simulink model "model_sim_CHB5_36_new_temp"  (R2020a)
settings: Solver=FixedStepAuto  StartTime=0.0  StopTime=5  RelTol=1e-3
InitFcn:
  | sysinit
values from neighbouring files (symbols this model uses):
  C = 0.03    [sysinit.m]
  C_f = 0.625e-6    (= 6.25e-07)    [sysinit.m]
  f = 50    [sysinit.m]
  f_switch = 500    [sysinit.m]
  L = 0.004    [sysinit.m]
  L_f = 3e-6    (= 3e-06)    [sysinit.m]
  R = 1.2    [sysinit.m]
  R_f = 1.5    [sysinit.m]
  Rth_h = 7.5e-3    (= 0.0075)    [Device_Parameter.m]
  Rth_h_tau = 0.5    [Device_Parameter.m]
  st = 5e-7    (= 5e-07)    [sysinit.m]
  temp_init = 40    [sysinit.m]
  Ts = 1e-6    (= 1e-06)    [sysinit.m]
  Ts2 = 0.5E-3    (= 0.0005)    [sysinit.m]
  Udc = 2500    [sysinit.m]
undefined symbols (not defined in the file or in its folder): DIODE_204520, DIODE_344520, DIODE_D1031SH, DIODE_D1331SH, IGCT_364520_36, IGCT_364521_36, IGCT_654522_6, magnitude, Ts1
libraries: powerlib x278, powerlib_meascontrol x84, simulink x9
(part 1 of 5)
settings Model: SimulationMode=accelerator  Creator=jhchen  LastModifiedBy=Jhchen
settings DataIOCC: ReturnWorkspaceOutputs=off
settings DebuggingCC: UnconnectedInputMsg=none  UnconnectedOutputMsg=none  UnconnectedLineMsg=none
settings ModelReferenceCC: EnableRefExpFcnMdlSchedulingChecks=off
settings RTWCC: Description=Generic Real-Time Target

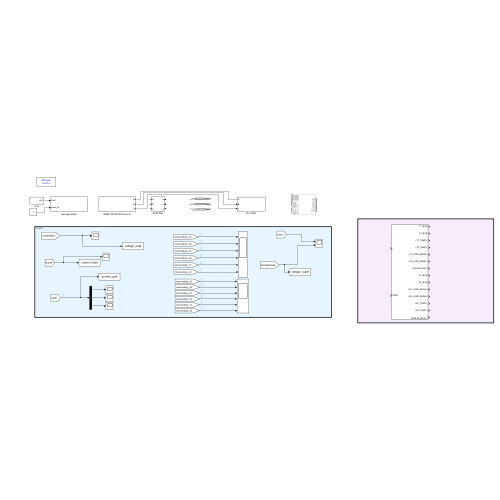
[thumbnail: Simulink's stored preview of the top-level diagram]
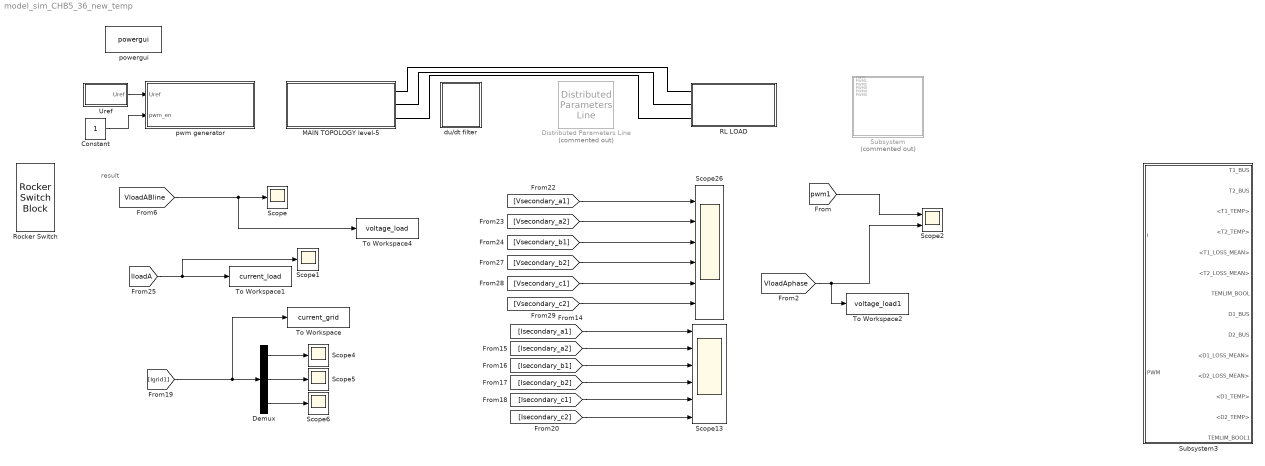
== system model_sim_CHB5_36_new_temp ==
  note: result
  Constant : Constant  OutDataTypeStr=boolean
  Demux : Demux  Outputs=3
  Distributed Parameters Line : powerlib/Elements/Distributed Parameters Line  Commented=on  Phases=3  Length=150e-3  Frequency=60  Resistance=[0.01273 0.3864]  Inductance="[0.9337e-3  4.1264e-3]"  Capacitance=[12.74e-9 7.751e-9]  x1=[0 0 0 0; 0.0001244 0 0 0; 0.0002488 0 0 0; 0.0003733 0 0 0; 0.0004977 0 0 0; 0.0006221 0 0 0]  x2=[0 0 0 0; 0.0001244 0 0 0; 0.0002488 0 0 0; 0.0003733 0 0 0; 0.0004977 0 0 0; 0.0006221 0 0 0]  x3=[0 0 0 0; 0.0001244 0 0 0; 0.0002488 0 0 0; 0.0003733 0 0 0; 0.0004977 0 0 0; 0.0006221 0 0 0]  x4=[0 0 0 0; 0.0001244 0 0 0; 0.0002488 0 0 0; 0.0003733 0 0 0; 0.0004977 0 0 0; 0.0006221 0 0 0]  x5=0  V1=ones(3,3)  V2=ones(3,3)  I1=ones(3,3)  I2=ones(3,3)  nHarmo=1  Measurements=None  Decoupling=off  VsMag0=0  VrMag0=0  VsAngle0=0  VrAngle0=0  IsMag0=0  IrMag0=0  IsAngle0=0  IrAngle0=0
  MAIN TOPOLOGY level-5 : Subsystem
  RL LOAD : Subsystem
  Rocker Switch : RockerSwitchBlock
      settings: Values={{'Off', 'On'}, [0 1]}
  Scope{,1,4..6} (5 alike) : Scope
  Scope13 : Scope  NumInputPorts=6
  Scope2 : Scope  NumInputPorts=2
  Scope26 : Scope  NumInputPorts=6
  Subsystem : Subsystem  Commented=on
  Subsystem3 : Subsystem  mask{IGCTTP=65L4522, DIODE_TP=34L4520}
      mask prompts: IGCTTP "IGCT_DEVICE"; DIODE_TP "DIODE_DEVICE"
      mask TypeOptions IGCTTP: 36L4520 | 36L4521 | 65L4522
      mask TypeOptions DIODE_TP: 20L4520 | 34L4520 | D1031SH | D1331SH
      mask DialogControl ParameterGroupVar Prompt: DEVICE TYPE
  To Workspace : ToWorkspace  VariableName=current_grid  SaveFormat=Structure With Time  SampleTime=-1
  To Workspace1 : ToWorkspace  VariableName=current_load  SaveFormat=Structure With Time  SampleTime=-1
  To Workspace2 : ToWorkspace  VariableName=voltage_load1  SaveFormat=Structure With Time  SampleTime=-1
  To Workspace4 : ToWorkspace  VariableName=voltage_load  SaveFormat=Structure With Time  SampleTime=-1
  Uref : Subsystem  mask{m=1, f=f, nn=0, deg=0}
      mask prompts: m "m_p调制比"; f "f_module输出频率"; nn "电压增加百分量"; deg "电流移相角度"
      mask DialogControl ParameterGroupVar Prompt: 参数
  du/dt filter : Subsystem
  powergui : powerlib/powergui  Priority=1  SimulationMode=Discrete  SampleTime=st  frequency=60  Iterations=50  frequencyindice=50  Pbase=100e6  ErrMax=1e-4  UnitsV=kV  UnitsW=MW  buscounter=0  FunctionMessages=off  echomessages=off  EnableUseOfTLC=off  CurrentSourceSwitches=off  DisableSnubberDevices=off  DisableRonSwitches=off  DisableVfSwitches=off  DisplayEquations=off  AutomaticDiscreteSolvers=off  SolverType=Tustin/Backward Euler (TBE)  Interpol=off  ExternalGateDelay=off  methode=off  Ts=100  x0status=blocks  SPID=on  SwTol=0  HookPort=off  NonlinearTolerance=1e-4  nMaxIteration=100  ContinueOnMaxIteration=off  RestoreLinks=warning  ResistiveCurrentMeasurement=off  Frange=[0:2:500]  Ylog=off  Xlog=on  ShowGrid=off  save=off  variable=ZData  structure=0  ZoomFFT=off  StartTime=0.0  cycles=1  DisplayStyle=1  fundamental=60  FreqAxis=off  MaxFrequency=1000  frequencyindicesteady=1  RmsSteady=1  display=off
  pwm generator : Subsystem  mask{f_car=f_switch, tt=1/4, ttd=0}
      mask prompts: f_car "f_carrier载波频率"; tt "ts载波移相周期"; ttd "td防直通延时"
      mask DialogControl ParameterGroupVar Prompt: 参数
  wires:
  Uref/1(Uref) -> pwm generator/1(Uref)
  [Isecondary_c2] -> Scope13/6
  [Isecondary_b2] -> Scope13/4
  [Isecondary_a2] -> Scope13/2
  Demux/2 -> Scope5/1
  [Vsecondary_b2] -> Scope26/4
  [Vsecondary_b1] -> Scope26/3
  [Isecondary_c1] -> Scope13/5
  [Vsecondary_a1] -> Scope26/1
  Demux/1 -> Scope4/1
  [Isecondary_a1] -> Scope13/1
  Demux/3 -> Scope6/1
  [Vsecondary_c2] -> Scope26/6
  [Igrid1] -> Demux/1, To Workspace/1
  [IloadA] -> Scope1/1, To Workspace1/1
  [Isecondary_b1] -> Scope13/3
  [Vsecondary_c1] -> Scope26/5
  [VloadABline] -> To Workspace4/1, Scope/1
  [Vsecondary_a2] -> Scope26/2
  [pwm1] -> Scope2/1
  [VloadAphase] -> To Workspace2/1, Scope2/2
  Constant/1 -> pwm generator/2(pwm_en)
  connections:
  RL LOAD/LConn1 -- MAIN TOPOLOGY level-5/RConn1
  RL LOAD/LConn2 -- MAIN TOPOLOGY level-5/RConn2
  RL LOAD/LConn3 -- MAIN TOPOLOGY level-5/RConn3

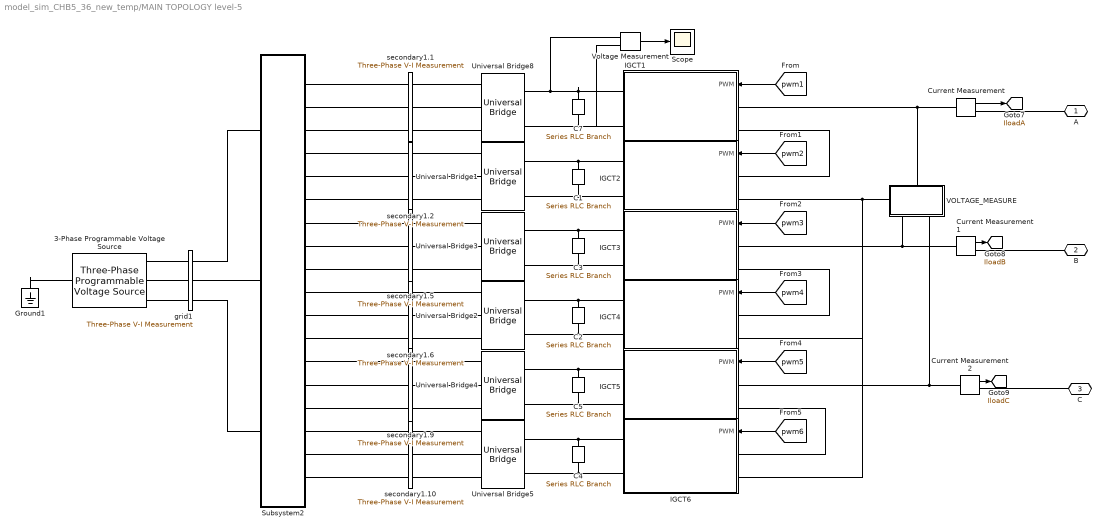
== system model_sim_CHB5_36_new_temp/MAIN TOPOLOGY level-5 ==
  3-Phase Programmable Voltage Source : powerlib/Electrical Sources/Three-Phase Programmable Voltage Source  PositiveSequence=[10000 0 50]  VariationEntity=None  VariationType=Step  VariationTypeAlt=Step  VariationStep=0.5  VariationRate=10  VariationMagnitude=0.3  VariationFrequency=2  VariationTiming=[0.05 1]  VariationPhaseA=off  Amplitudes=[1 0.8 1.2 1.0]  TimeValues=[0 0.1 0.15 0.2]  HarmonicGeneration=off  HarmonicA=[5 0.08 -45 2]  HarmonicB=[2 0 0 2]  Timing="[0.1  1]"  BusType=swing  Pref=0  Qref=0  Qmin=-inf  Qmax=inf
  C{1..5,7} (6 alike) : powerlib/Elements/Series RLC Branch  LConnTagsString=__new0  RConnTagsString=__new0  BranchType=C  Resistance=0.0001  Inductance=1.0  SetiL0=off  InitialCurrent=0  Capacitance=C  Setx0=on  InitialVoltage=2500  Measurements=None
  Current Measurement : powerlib/Measurements/Current Measurement  PhasorSimulation=off  OutputType=Complex  PSBequivalent=0
  Current Measurement1 : powerlib/Measurements/Current Measurement  PhasorSimulation=off  OutputType=Complex  PSBequivalent=0
  Current Measurement2 : powerlib/Measurements/Current Measurement  PhasorSimulation=off  OutputType=Complex  PSBequivalent=0
  Ground1 : powerlib/Elements/Ground  LConnTagsString=a
  IGCT1 : Subsystem
      settings: PortSchema="{\"entries\":[{\"content\":{\"sides\":[{\"content\":{\"connectorIds\":[\"LConn1\",\"LConn2\"]},\"type\":\"ConnectorPlacement.EquallySpacedRectSide\",\"uuid\":\"3b5227fd-32cc-4097-9a6a-2909540651e9\"},{\"content\":{\"connectorIds\":[\"In1\",\"RConn1\",\"RConn2\"],\"side\":\"RIGHT\"},\"type\":\"ConnectorPlacement.EquallySpacedRectSide\",\"uuid\":\"b0068562-9d9a-456b-acd2-db870c5bcace\"},{\"content\":{\"side\":\"TOP\"},\"type\":\"ConnectorPlacement.EquallySpacedRectSide\",\"uuid\":\"bbecbe08-a8e7-4703-9f6f-443f87d924da\"}]},\"type\":\"ConnectorPlacement.EquallySpacedConnector\",\"uuid\":\"6ec83c7b-e3bb-4502-bc8f-4da9ff103a20\"}],\"packageUris\":[\"http://schema.mathworks.com/mf0/Connector/R2020b\"],\"version\":\"1.0\"}"
  IGCT2 : Subsystem
      settings: PortSchema="{\"entries\":[{\"content\":{\"sides\":[{\"content\":{\"connectorIds\":[\"LConn1\",\"LConn2\"]},\"type\":\"ConnectorPlacement.EquallySpacedRectSide\",\"uuid\":\"3b5227fd-32cc-4097-9a6a-2909540651e9\"},{\"content\":{\"connectorIds\":[\"In1\",\"RConn1\",\"RConn2\"],\"side\":\"RIGHT\"},\"type\":\"ConnectorPlacement.EquallySpacedRectSide\",\"uuid\":\"b0068562-9d9a-456b-acd2-db870c5bcace\"},{\"content\":{\"side\":\"TOP\"},\"type\":\"ConnectorPlacement.EquallySpacedRectSide\",\"uuid\":\"bbecbe08-a8e7-4703-9f6f-443f87d924da\"}]},\"type\":\"ConnectorPlacement.EquallySpacedConnector\",\"uuid\":\"6ec83c7b-e3bb-4502-bc8f-4da9ff103a20\"}],\"packageUris\":[\"http://schema.mathworks.com/mf0/Connector/R2020b\"],\"version\":\"1.0\"}"
  IGCT3 : Subsystem
      settings: PortSchema="{\"entries\":[{\"content\":{\"sides\":[{\"content\":{\"connectorIds\":[\"LConn1\",\"LConn2\"]},\"type\":\"ConnectorPlacement.EquallySpacedRectSide\",\"uuid\":\"3b5227fd-32cc-4097-9a6a-2909540651e9\"},{\"content\":{\"connectorIds\":[\"In1\",\"RConn1\",\"RConn2\"],\"side\":\"RIGHT\"},\"type\":\"ConnectorPlacement.EquallySpacedRectSide\",\"uuid\":\"b0068562-9d9a-456b-acd2-db870c5bcace\"},{\"content\":{\"side\":\"TOP\"},\"type\":\"ConnectorPlacement.EquallySpacedRectSide\",\"uuid\":\"bbecbe08-a8e7-4703-9f6f-443f87d924da\"}]},\"type\":\"ConnectorPlacement.EquallySpacedConnector\",\"uuid\":\"6ec83c7b-e3bb-4502-bc8f-4da9ff103a20\"}],\"packageUris\":[\"http://schema.mathworks.com/mf0/Connector/R2020b\"],\"version\":\"1.0\"}"
  IGCT4 : Subsystem
      settings: PortSchema="{\"entries\":[{\"content\":{\"sides\":[{\"content\":{\"connectorIds\":[\"LConn1\",\"LConn2\"]},\"type\":\"ConnectorPlacement.EquallySpacedRectSide\",\"uuid\":\"3b5227fd-32cc-4097-9a6a-2909540651e9\"},{\"content\":{\"connectorIds\":[\"In1\",\"RConn1\",\"RConn2\"],\"side\":\"RIGHT\"},\"type\":\"ConnectorPlacement.EquallySpacedRectSide\",\"uuid\":\"b0068562-9d9a-456b-acd2-db870c5bcace\"},{\"content\":{\"side\":\"TOP\"},\"type\":\"ConnectorPlacement.EquallySpacedRectSide\",\"uuid\":\"bbecbe08-a8e7-4703-9f6f-443f87d924da\"}]},\"type\":\"ConnectorPlacement.EquallySpacedConnector\",\"uuid\":\"6ec83c7b-e3bb-4502-bc8f-4da9ff103a20\"}],\"packageUris\":[\"http://schema.mathworks.com/mf0/Connector/R2020b\"],\"version\":\"1.0\"}"
  IGCT5 : Subsystem
      settings: PortSchema="{\"entries\":[{\"content\":{\"sides\":[{\"content\":{\"connectorIds\":[\"LConn1\",\"LConn2\"]},\"type\":\"ConnectorPlacement.EquallySpacedRectSide\",\"uuid\":\"3b5227fd-32cc-4097-9a6a-2909540651e9\"},{\"content\":{\"connectorIds\":[\"In1\",\"RConn1\",\"RConn2\"],\"side\":\"RIGHT\"},\"type\":\"ConnectorPlacement.EquallySpacedRectSide\",\"uuid\":\"b0068562-9d9a-456b-acd2-db870c5bcace\"},{\"content\":{\"side\":\"TOP\"},\"type\":\"ConnectorPlacement.EquallySpacedRectSide\",\"uuid\":\"bbecbe08-a8e7-4703-9f6f-443f87d924da\"}]},\"type\":\"ConnectorPlacement.EquallySpacedConnector\",\"uuid\":\"6ec83c7b-e3bb-4502-bc8f-4da9ff103a20\"}],\"packageUris\":[\"http://schema.mathworks.com/mf0/Connector/R2020b\"],\"version\":\"1.0\"}"
  IGCT6 : Subsystem
      settings: PortSchema="{\"entries\":[{\"content\":{\"sides\":[{\"content\":{\"connectorIds\":[\"LConn1\",\"LConn2\"]},\"type\":\"ConnectorPlacement.EquallySpacedRectSide\",\"uuid\":\"3b5227fd-32cc-4097-9a6a-2909540651e9\"},{\"content\":{\"connectorIds\":[\"In1\",\"RConn1\",\"RConn2\"],\"side\":\"RIGHT\"},\"type\":\"ConnectorPlacement.EquallySpacedRectSide\",\"uuid\":\"b0068562-9d9a-456b-acd2-db870c5bcace\"},{\"content\":{\"side\":\"TOP\"},\"type\":\"ConnectorPlacement.EquallySpacedRectSide\",\"uuid\":\"bbecbe08-a8e7-4703-9f6f-443f87d924da\"}]},\"type\":\"ConnectorPlacement.EquallySpacedConnector\",\"uuid\":\"6ec83c7b-e3bb-4502-bc8f-4da9ff103a20\"}],\"packageUris\":[\"http://schema.mathworks.com/mf0/Connector/R2020b\"],\"version\":\"1.0\"}"
  Scope : Scope
  Subsystem2 : Subsystem  mask{p=4e6, vp=10000/6, vs=1900, windingpri=[0.0125 0.01], windingsec=[0.0125  0.08], mag=[500  500]}
      mask prompts: p "Nominal power"; vp "Primary nominal voltage Vp (VrmsPh-Ph)"; vs "Scecondary nominal voltage"; windingpri "Winding primary [R L]"; windingsec "Winding secondary [R L]"; mag "Magnetizing branch [Rm Lm]"
      mask DialogControl ParameterGroupVar Prompt: 参数
  Universal Bridge{1..5,8} (6 alike) : powerlib/Power Electronics/Universal Bridge  Arms=3  SnubberResistance=1e5  SnubberCapacitance=inf  Device=Diodes  Ron=1e-3  Lon=0  ForwardVoltages="[  0  0  ]"  ForwardVoltage=0  GTOparameters=[ 10e-6 , 20e-6 ]  IGBTparameters=[ 1e-6 , 2e-6 ]  Measurements=All voltages and currents  Measurements_2=None  converterType=Rectifier
  VOLTAGE_MEASURE : Subsystem
      settings: PortSchema="{\"entries\":[{\"content\":{\"sides\":[{\"content\":{\"connectorIds\":[\"LConn1\"]},\"type\":\"ConnectorPlacement.EquallySpacedRectSide\",\"uuid\":\"e0cdf748-1c1e-4377-bca6-4a33d23f4a26\"},{\"content\":{\"side\":\"RIGHT\"},\"type\":\"ConnectorPlacement.EquallySpacedRectSide\",\"uuid\":\"7345d1e9-e146-4d05-bc9d-06c5f4bfd43e\"},{\"content\":{\"connectorIds\":[\"LConn2\"],\"side\":\"TOP\"},\"type\":\"ConnectorPlacement.EquallySpacedRectSide\",\"uuid\":\"2ef5394b-e3d5-43ec-bd76-ec9d8d58d678\"},{\"content\":{\"connectorIds\":[\"RConn1\",\"RConn2\"],\"side\":\"BOTTOM\"},\"type\":\"ConnectorPlacement.EquallySpacedRectSide\",\"uuid\":\"2dd50293-b78e-4e40-a029-347d4d381fe9\"}]},\"type\":\"ConnectorPlacement.EquallySpacedConnector\",\"uuid\":\"a79e479b-e54c-4d34-8e2f-a0f7c0fb898b\"}],\"packageUris\":[\"http://schema.mathworks.com/mf0/Connector/R2020b\"],\"version\":\"1.0\"}"
  Voltage Measurement : powerlib/Measurements/Voltage Measurement  PhasorSimulation=off  OutputType=Complex  PSBequivalent=0
  grid1 : powerlib/Measurements/Three-Phase V-I Measurement  VoltageMeasurement=phase-to-ground  SetLabelV=on  LabelV=Vgrid1  Vpu=off  VpuLL=off  CurrentMeasurement=yes  SetLabelI=on  LabelI=Igrid1  Ipu=off  Pbase=1e3  Vbase=380  OutputType=Magnitude  PhasorSimulation=off  PSBequivalent=0
  secondary1.1 : powerlib/Measurements/Three-Phase V-I Measurement  VoltageMeasurement=phase-to-phase  SetLabelV=on  LabelV=Vsecondary_a1  Vpu=off  VpuLL=off  CurrentMeasurement=yes  SetLabelI=on  LabelI=Isecondary_a1  Ipu=off  Pbase=1e3  Vbase=380  OutputType=Magnitude  PhasorSimulation=off  PSBequivalent=0
  secondary1.10 : powerlib/Measurements/Three-Phase V-I Measurement  VoltageMeasurement=phase-to-phase  SetLabelV=on  LabelV=Vsecondary_c2  Vpu=off  VpuLL=off  CurrentMeasurement=yes  SetLabelI=on  LabelI=Isecondary_c2  Ipu=off  Pbase=1e3  Vbase=380  OutputType=Magnitude  PhasorSimulation=off  PSBequivalent=0
  secondary1.2 : powerlib/Measurements/Three-Phase V-I Measurement  VoltageMeasurement=phase-to-phase  SetLabelV=on  LabelV=Vsecondary_a2  Vpu=off  VpuLL=off  CurrentMeasurement=yes  SetLabelI=on  LabelI=Isecondary_a2  Ipu=off  Pbase=1e3  Vbase=380  OutputType=Magnitude  PhasorSimulation=off  PSBequivalent=0
  secondary1.5 : powerlib/Measurements/Three-Phase V-I Measurement  VoltageMeasurement=phase-to-phase  SetLabelV=on  LabelV=Vsecondary_b1  Vpu=off  VpuLL=off  CurrentMeasurement=yes  SetLabelI=on  LabelI=Isecondary_b1  Ipu=off  Pbase=1e3  Vbase=380  OutputType=Magnitude  PhasorSimulation=off  PSBequivalent=0
  secondary1.6 : powerlib/Measurements/Three-Phase V-I Measurement  VoltageMeasurement=phase-to-phase  SetLabelV=on  LabelV=Vsecondary_b2  Vpu=off  VpuLL=off  CurrentMeasurement=yes  SetLabelI=on  LabelI=Isecondary_b2  Ipu=off  Pbase=1e3  Vbase=380  OutputType=Magnitude  PhasorSimulation=off  PSBequivalent=0
  secondary1.9 : powerlib/Measurements/Three-Phase V-I Measurement  VoltageMeasurement=phase-to-phase  SetLabelV=on  LabelV=Vsecondary_c1  Vpu=off  VpuLL=off  CurrentMeasurement=yes  SetLabelI=on  LabelI=Isecondary_c1  Ipu=off  Pbase=1e3  Vbase=380  OutputType=Magnitude  PhasorSimulation=off  PSBequivalent=0
  A : PMIOPort  Side=Right
  B : PMIOPort  Port=2  Side=Right
  C : PMIOPort  Port=3  Side=Right
  tag scope: IloadA=global, IloadB=global, IloadC=global
  wires:
  [pwm1] -> IGCT1/1(PWM)
  Current Measurement2/1 -> [IloadC]
  [pwm2] -> IGCT2/1(PWM)
  [pwm5] -> IGCT5/1(PWM)
  [pwm6] -> IGCT6/1(PWM)
  [pwm4] -> IGCT4/1(PWM)
  [pwm3] -> IGCT3/1(PWM)
  Current Measurement1/1 -> [IloadB]
  Current Measurement/1 -> [IloadA]
  Voltage Measurement/1 -> Scope/1
  connections:
  Subsystem2/RConn7 -- secondary1.5/LConn1
  Universal Bridge5/RConn1 -- IGCT6/LConn1 -- C4/LConn1
  Universal Bridge4/LConn2 -- secondary1.9/RConn2
  Current Measurement2/LConn1 -- IGCT5/RConn1 -- VOLTAGE_MEASURE/RConn2
  secondary1.2/RConn1 -- Universal Bridge1/LConn1
  Universal Bridge5/LConn2 -- secondary1.10/RConn2
  Universal Bridge3/RConn1 -- IGCT3/LConn1 -- C3/LConn1
  Subsystem2/RConn5 -- secondary1.2/LConn2
  Ground1/LConn1 -- 3-Phase Programmable Voltage Source/LConn1
  Subsystem2/RConn16 -- secondary1.10/LConn1
  Subsystem2/RConn14 -- secondary1.9/LConn2
  Subsystem2/RConn3 -- secondary1.1/LConn3
  Subsystem2/RConn6 -- secondary1.2/LConn3
  Universal Bridge4/RConn2 -- IGCT5/LConn2 -- C5/RConn1
  Universal Bridge1/RConn1 -- C1/LConn1 -- IGCT2/LConn1
  Current Measurement/LConn1 -- IGCT1/RConn1 -- VOLTAGE_MEASURE/LConn2
  Universal Bridge3/RConn2 -- IGCT3/LConn2 -- C3/RConn1
  Universal Bridge2/RConn1 -- IGCT4/LConn1 -- C2/LConn1
  C7/LConn1 -- IGCT1/LConn1 -- Voltage Measurement/LConn1 -- Universal Bridge8/RConn1
  Universal Bridge1/RConn2 -- IGCT2/LConn2 -- C1/RConn1
  Subsystem2/RConn12 -- secondary1.6/LConn3
  Subsystem2/LConn2 -- grid1/RConn2
  Subsystem2/LConn3 -- grid1/RConn3
  Current Measurement1/LConn1 -- IGCT3/RConn1 -- VOLTAGE_MEASURE/RConn1
  IGCT4/RConn1 -- IGCT3/RConn2
  Subsystem2/RConn15 -- secondary1.9/LConn3
  Universal Bridge5/RConn2 -- IGCT6/LConn2 -- C4/RConn1
  secondary1.2/RConn2 -- Universal Bridge1/LConn2
  C7/RConn1 -- Voltage Measurement/LConn2 -- IGCT1/LConn2 -- Universal Bridge8/RConn2
  secondary1.6/RConn2 -- Universal Bridge2/LConn2
  Universal Bridge4/LConn3 -- secondary1.9/RConn3
  Subsystem2/RConn1 -- secondary1.1/LConn1
  secondary1.1/RConn2 -- Universal Bridge8/LConn2
  grid1/LConn1 -- 3-Phase Programmable Voltage Source/RConn1
  Subsystem2/RConn10 -- secondary1.6/LConn1
  secondary1.1/RConn3 -- Universal Bridge8/LConn3
  grid1/LConn2 -- 3-Phase Programmable Voltage Source/RConn2
  Universal Bridge5/LConn3 -- secondary1.10/RConn3
  Universal Bridge4/LConn1 -- secondary1.9/RConn1
  Universal Bridge5/LConn1 -- secondary1.10/RConn1
  grid1/LConn3 -- 3-Phase Programmable Voltage Source/RConn3
  secondary1.1/RConn1 -- Universal Bridge8/LConn1
  Subsystem2/RConn2 -- secondary1.1/LConn2
  Subsystem2/RConn4 -- secondary1.2/LConn1
  Subsystem2/LConn1 -- grid1/RConn1
  secondary1.6/RConn1 -- Universal Bridge2/LConn1
  secondary1.6/RConn3 -- Universal Bridge2/LConn3
  Universal Bridge2/RConn2 -- IGCT4/LConn2 -- C2/RConn1
  Subsystem2/RConn18 -- secondary1.10/LConn3
  Subsystem2/RConn13 -- secondary1.9/LConn1
  Subsystem2/RConn9 -- secondary1.5/LConn3
  Subsystem2/RConn11 -- secondary1.6/LConn2
  Subsystem2/RConn8 -- secondary1.5/LConn2
  Subsystem2/RConn17 -- secondary1.10/LConn2
  Universal Bridge4/RConn1 -- IGCT5/LConn1 -- C5/LConn1
  IGCT6/RConn1 -- IGCT5/RConn2
  IGCT2/RConn1 -- IGCT1/RConn2
  secondary1.5/RConn2 -- Universal Bridge3/LConn2
  secondary1.5/RConn3 -- Universal Bridge3/LConn3
  secondary1.5/RConn1 -- Universal Bridge3/LConn1
  secondary1.2/RConn3 -- Universal Bridge1/LConn3
  Current Measurement2/RConn1 -- C/RConn1
  Current Measurement/RConn1 -- A/RConn1
  B/RConn1 -- Current Measurement1/RConn1
  IGCT6/RConn2 -- IGCT4/RConn2 -- IGCT2/RConn2 -- VOLTAGE_MEASURE/LConn1

== system model_sim_CHB5_36_new_temp/RL LOAD ==
  Scope : Scope  NumInputPorts=2
  Series RLC Branch1 : powerlib/Elements/Series RLC Branch  LConnTagsString=__new0  RConnTagsString=__new0  BranchType=RL  Resistance=R  Inductance=L  SetiL0=off  InitialCurrent=0  Capacitance=1e-6  Setx0=off  InitialVoltage=0  Measurements=None
  Series RLC Branch2 : powerlib/Elements/Series RLC Branch  LConnTagsString=__new0  RConnTagsString=__new0  BranchType=RL  Resistance=R  Inductance=L  SetiL0=off  InitialCurrent=0  Capacitance=1e-6  Setx0=off  InitialVoltage=0  Measurements=None
  Series RLC Branch7 : powerlib/Elements/Series RLC Branch  LConnTagsString=__new0  RConnTagsString=__new0  BranchType=RL  Resistance=R  Inductance=L  SetiL0=off  InitialCurrent=0  Capacitance=1e-6  Setx0=off  InitialVoltage=0  Measurements=None
  Voltage Measurement : powerlib/Measurements/Voltage Measurement  PhasorSimulation=off  OutputType=Complex  PSBequivalent=0
  A : PMIOPort  Side=Left
  B : PMIOPort  Port=2  Side=Left
  C : PMIOPort  Port=3  Side=Left
  wires:
  Voltage Measurement/1 -> Scope/2
  [VloadAphase] -> Scope/1
  connections:
  Series RLC Branch7/RConn1 -- Series RLC Branch2/RConn1 -- Series RLC Branch1/RConn1 -- Voltage Measurement/LConn2
  Series RLC Branch2/LConn1 -- C/RConn1
  Series RLC Branch7/LConn1 -- Voltage Measurement/LConn1 -- A/RConn1
  Series RLC Branch1/LConn1 -- B/RConn1

== system model_sim_CHB5_36_new_temp/Subsystem ==
  PWM : Inport
  PWM1 : Inport  Port=2
  PWM2 : Inport  Port=3
  PWM3 : Inport  Port=4
  PWM4 : Inport  Port=5
  PWM5 : Inport  Port=6
  IGCT1 : Subsystem
      settings: PortSchema="{\"entries\":[{\"content\":{\"sides\":[{\"content\":{\"connectorIds\":[\"LConn1\",\"LConn2\"]},\"type\":\"ConnectorPlacement.EquallySpacedRectSide\",\"uuid\":\"3b5227fd-32cc-4097-9a6a-2909540651e9\"},{\"content\":{\"connectorIds\":[\"In1\",\"RConn1\",\"RConn2\"],\"side\":\"RIGHT\"},\"type\":\"ConnectorPlacement.EquallySpacedRectSide\",\"uuid\":\"b0068562-9d9a-456b-acd2-db870c5bcace\"},{\"content\":{\"side\":\"TOP\"},\"type\":\"ConnectorPlacement.EquallySpacedRectSide\",\"uuid\":\"bbecbe08-a8e7-4703-9f6f-443f87d924da\"},{\"content\":{\"side\":\"BOTTOM\"},\"type\":\"ConnectorPlacement.EquallySpacedRectSide\",\"uuid\":\"38988ce8-647b-48d0-a974-68b7c64b6edd\"}]},\"type\":\"ConnectorPlacement.EquallySpacedConnector\",\"uuid\":\"6ec83c7b-e3bb-4502-bc8f-4da9ff103a20\"}],\"packageUris\":[\"http://schema.mathworks.com/mf0/Connector/R2020b\"],\"version\":\"1.0\"}"
  IGCT2 : Subsystem
      settings: PortSchema="{\"entries\":[{\"content\":{\"sides\":[{\"content\":{\"connectorIds\":[\"LConn1\",\"LConn2\"]},\"type\":\"ConnectorPlacement.EquallySpacedRectSide\",\"uuid\":\"3b5227fd-32cc-4097-9a6a-2909540651e9\"},{\"content\":{\"connectorIds\":[\"In1\",\"RConn1\",\"RConn2\"],\"side\":\"RIGHT\"},\"type\":\"ConnectorPlacement.EquallySpacedRectSide\",\"uuid\":\"b0068562-9d9a-456b-acd2-db870c5bcace\"},{\"content\":{\"side\":\"TOP\"},\"type\":\"ConnectorPlacement.EquallySpacedRectSide\",\"uuid\":\"bbecbe08-a8e7-4703-9f6f-443f87d924da\"},{\"content\":{\"side\":\"BOTTOM\"},\"type\":\"ConnectorPlacement.EquallySpacedRectSide\",\"uuid\":\"38988ce8-647b-48d0-a974-68b7c64b6edd\"}]},\"type\":\"ConnectorPlacement.EquallySpacedConnector\",\"uuid\":\"6ec83c7b-e3bb-4502-bc8f-4da9ff103a20\"}],\"packageUris\":[\"http://schema.mathworks.com/mf0/Connector/R2020b\"],\"version\":\"1.0\"}"
  IGCT3 : Subsystem
      settings: PortSchema="{\"entries\":[{\"content\":{\"sides\":[{\"content\":{\"connectorIds\":[\"LConn1\",\"LConn2\"]},\"type\":\"ConnectorPlacement.EquallySpacedRectSide\",\"uuid\":\"3b5227fd-32cc-4097-9a6a-2909540651e9\"},{\"content\":{\"connectorIds\":[\"In1\",\"RConn1\",\"RConn2\"],\"side\":\"RIGHT\"},\"type\":\"ConnectorPlacement.EquallySpacedRectSide\",\"uuid\":\"b0068562-9d9a-456b-acd2-db870c5bcace\"},{\"content\":{\"side\":\"TOP\"},\"type\":\"ConnectorPlacement.EquallySpacedRectSide\",\"uuid\":\"bbecbe08-a8e7-4703-9f6f-443f87d924da\"},{\"content\":{\"side\":\"BOTTOM\"},\"type\":\"ConnectorPlacement.EquallySpacedRectSide\",\"uuid\":\"38988ce8-647b-48d0-a974-68b7c64b6edd\"}]},\"type\":\"ConnectorPlacement.EquallySpacedConnector\",\"uuid\":\"6ec83c7b-e3bb-4502-bc8f-4da9ff103a20\"}],\"packageUris\":[\"http://schema.mathworks.com/mf0/Connector/R2020b\"],\"version\":\"1.0\"}"
  IGCT4 : Subsystem
      settings: PortSchema="{\"entries\":[{\"content\":{\"sides\":[{\"content\":{\"connectorIds\":[\"LConn1\",\"LConn2\"]},\"type\":\"ConnectorPlacement.EquallySpacedRectSide\",\"uuid\":\"3b5227fd-32cc-4097-9a6a-2909540651e9\"},{\"content\":{\"connectorIds\":[\"In1\",\"RConn1\",\"RConn2\"],\"side\":\"RIGHT\"},\"type\":\"ConnectorPlacement.EquallySpacedRectSide\",\"uuid\":\"b0068562-9d9a-456b-acd2-db870c5bcace\"},{\"content\":{\"side\":\"TOP\"},\"type\":\"ConnectorPlacement.EquallySpacedRectSide\",\"uuid\":\"bbecbe08-a8e7-4703-9f6f-443f87d924da\"},{\"content\":{\"side\":\"BOTTOM\"},\"type\":\"ConnectorPlacement.EquallySpacedRectSide\",\"uuid\":\"38988ce8-647b-48d0-a974-68b7c64b6edd\"}]},\"type\":\"ConnectorPlacement.EquallySpacedConnector\",\"uuid\":\"6ec83c7b-e3bb-4502-bc8f-4da9ff103a20\"}],\"packageUris\":[\"http://schema.mathworks.com/mf0/Connector/R2020b\"],\"version\":\"1.0\"}"
  IGCT5 : Subsystem
      settings: PortSchema="{\"entries\":[{\"content\":{\"sides\":[{\"content\":{\"connectorIds\":[\"LConn1\",\"LConn2\"]},\"type\":\"ConnectorPlacement.EquallySpacedRectSide\",\"uuid\":\"3b5227fd-32cc-4097-9a6a-2909540651e9\"},{\"content\":{\"connectorIds\":[\"In1\",\"RConn1\",\"RConn2\"],\"side\":\"RIGHT\"},\"type\":\"ConnectorPlacement.EquallySpacedRectSide\",\"uuid\":\"b0068562-9d9a-456b-acd2-db870c5bcace\"},{\"content\":{\"side\":\"TOP\"},\"type\":\"ConnectorPlacement.EquallySpacedRectSide\",\"uuid\":\"bbecbe08-a8e7-4703-9f6f-443f87d924da\"},{\"content\":{\"side\":\"BOTTOM\"},\"type\":\"ConnectorPlacement.EquallySpacedRectSide\",\"uuid\":\"38988ce8-647b-48d0-a974-68b7c64b6edd\"}]},\"type\":\"ConnectorPlacement.EquallySpacedConnector\",\"uuid\":\"6ec83c7b-e3bb-4502-bc8f-4da9ff103a20\"}],\"packageUris\":[\"http://schema.mathworks.com/mf0/Connector/R2020b\"],\"version\":\"1.0\"}"
  IGCT6 : Subsystem
      settings: PortSchema="{\"entries\":[{\"content\":{\"sides\":[{\"content\":{\"connectorIds\":[\"LConn1\",\"LConn2\"]},\"type\":\"ConnectorPlacement.EquallySpacedRectSide\",\"uuid\":\"3b5227fd-32cc-4097-9a6a-2909540651e9\"},{\"content\":{\"connectorIds\":[\"In1\",\"RConn1\",\"RConn2\"],\"side\":\"RIGHT\"},\"type\":\"ConnectorPlacement.EquallySpacedRectSide\",\"uuid\":\"b0068562-9d9a-456b-acd2-db870c5bcace\"},{\"content\":{\"side\":\"TOP\"},\"type\":\"ConnectorPlacement.EquallySpacedRectSide\",\"uuid\":\"bbecbe08-a8e7-4703-9f6f-443f87d924da\"},{\"content\":{\"side\":\"BOTTOM\"},\"type\":\"ConnectorPlacement.EquallySpacedRectSide\",\"uuid\":\"38988ce8-647b-48d0-a974-68b7c64b6edd\"}]},\"type\":\"ConnectorPlacement.EquallySpacedConnector\",\"uuid\":\"6ec83c7b-e3bb-4502-bc8f-4da9ff103a20\"}],\"packageUris\":[\"http://schema.mathworks.com/mf0/Connector/R2020b\"],\"version\":\"1.0\"}"
  Udc+ : PMIOPort  Side=Left
  p1 : PMIOPort  Port=2  Side=Right
  udc- : PMIOPort  Port=3  Side=Left
  p2 : PMIOPort  Port=4  Side=Right
  Udc+1 : PMIOPort  Port=5  Side=Left
  p3 : PMIOPort  Port=6  Side=Right
  udc-1 : PMIOPort  Port=7  Side=Left
  p4 : PMIOPort  Port=8  Side=Right
  Udc+2 : PMIOPort  Port=9  Side=Left
  p5 : PMIOPort  Port=10  Side=Right
  udc-2 : PMIOPort  Port=11  Side=Left
  p6 : PMIOPort  Port=12  Side=Right
  Udc+3 : PMIOPort  Port=13  Side=Left
  p7 : PMIOPort  Port=14  Side=Right
  udc-3 : PMIOPort  Port=15  Side=Left
  p8 : PMIOPort  Port=16  Side=Right
  Udc+4 : PMIOPort  Port=17  Side=Left
  p9 : PMIOPort  Port=18  Side=Right
  udc-4 : PMIOPort  Port=19  Side=Left
  p10 : PMIOPort  Port=20  Side=Right
  Udc+5 : PMIOPort  Port=21  Side=Left
  p11 : PMIOPort  Port=22  Side=Right
  udc-5 : PMIOPort  Port=23  Side=Left
  p12 : PMIOPort  Port=24  Side=Right
  wires:
  PWM/1 -> IGCT1/1(PWM)
  PWM4/1 -> IGCT5/1(PWM)
  PWM3/1 -> IGCT4/1(PWM)
  PWM5/1 -> IGCT6/1(PWM)
  PWM1/1 -> IGCT2/1(PWM)
  PWM2/1 -> IGCT3/1(PWM)
  connections:
  IGCT5/LConn2 -- udc-4/RConn1
  IGCT6/LConn2 -- udc-5/RConn1
  IGCT6/RConn2 -- p12/RConn1
  IGCT6/RConn1 -- p11/RConn1
  IGCT1/LConn1 -- Udc+/RConn1
  IGCT1/LConn2 -- udc-/RConn1
  IGCT6/LConn1 -- Udc+5/RConn1
  IGCT1/RConn1 -- p1/RConn1
  IGCT5/RConn1 -- p9/RConn1
  IGCT2/LConn2 -- udc-1/RConn1
  IGCT3/RConn1 -- p5/RConn1
  IGCT3/RConn2 -- p6/RConn1
  IGCT3/LConn1 -- Udc+2/RConn1
  IGCT2/RConn1 -- p3/RConn1
  IGCT3/LConn2 -- udc-2/RConn1
  IGCT2/RConn2 -- p4/RConn1
  IGCT4/LConn1 -- Udc+3/RConn1
  IGCT4/LConn2 -- udc-3/RConn1
  IGCT5/RConn2 -- p10/RConn1
  IGCT5/LConn1 -- Udc+4/RConn1
  IGCT4/RConn1 -- p7/RConn1
  IGCT4/RConn2 -- p8/RConn1
  IGCT1/RConn2 -- p2/RConn1
  IGCT2/LConn1 -- Udc+1/RConn1

== system model_sim_CHB5_36_new_temp/Subsystem3 ==
  i : Inport
  PWM : Inport  Port=2
  DIODE : Subsystem  Variant=on
  Demux : Demux
  IGCT : Subsystem  Variant=on  VariantControl=Variant Subsystem
  T1_BUS : Outport
  T2_BUS : Outport  Port=2
  <T1_TEMP> : Outport  Port=3
  <T2_TEMP> : Outport  Port=4
  <T1_LOSS_MEAN> : Outport  Port=5
  <T2_LOSS_MEAN> : Outport  Port=6
  TEMLIM_BOOL : Outport  Port=7
  D1_BUS : Outport  Port=8
  D2_BUS : Outport  Port=9
  <D1_LOSS_MEAN> : Outport  Port=10
  <D2_LOSS_MEAN> : Outport  Port=11
  <D1_TEMP> : Outport  Port=12
  <D2_TEMP> : Outport  Port=13
  TEMLIM_BOOL1 : Outport  Port=14
  wires:
  IGCT/2(T2_BUS) -> T2_BUS/1
  DIODE/7(TEMLIM_BOOL) -> TEMLIM_BOOL1/1
  Demux/1 -> DIODE/2(PWM1), IGCT/2(PWM1)
  DIODE/2(D2_BUS) -> D2_BUS/1
  DIODE/3(D1_LOSS_MEAN) -> <D1_LOSS_MEAN>/1
  Demux/2 -> DIODE/3(PWM2), IGCT/3(PWM2)
  Demux/4 -> DIODE/5(PWM4)
  Demux/3 -> DIODE/4(PWM3)
  IGCT/3(<T1_TEMP>) -> <T1_TEMP>/1
  DIODE/6(D2_TEMP) -> <D2_TEMP>/1
  IGCT/1(T1_BUS) -> T1_BUS/1
  IGCT/4(<T2_TEMP>) -> <T2_TEMP>/1
  IGCT/5(<T1_LOSS_MEAN>) -> <T1_LOSS_MEAN>/1
  i/1 -> DIODE/1(I), IGCT/1(I)
  IGCT/6(<T2_LOSS_MEAN>) -> <T2_LOSS_MEAN>/1
  IGCT/7(TEMLIM_BOOL) -> TEMLIM_BOOL/1
  DIODE/5(D1_TEMP) -> <D1_TEMP>/1
  DIODE/4(D2_LOSS_MEAN) -> <D2_LOSS_MEAN>/1
  DIODE/1(D1_BUS) -> D1_BUS/1
  PWM/1 -> Demux/1

== system model_sim_CHB5_36_new_temp/Uref ==
  Mux : Mux  Inputs=3
  Saddle_Wave : Subsystem
  Sine Wave -2/3pi rad : Sin  Amplitude=m*1000*(1+nn)  Frequency=f*2*pi  Phase=-2/3*pi+deg*pi  SampleTime=0
  Sine Wave 0 rad : Sin  Amplitude=m*1000*(1+nn)  Frequency=f*2*pi  Phase=deg*pi  SampleTime=0
  Sine Wave 2/3pi rad : Sin  Amplitude=m*1000*(1+nn)  Frequency=f*2*pi  Phase=2/3*pi+deg*pi  SampleTime=0
  Uref : Outport
  wires:
  Sine Wave 2/3pi rad/1 -> Saddle_Wave/3(C)
  Saddle_Wave/2(b) -> Mux/2
  Saddle_Wave/1(a) -> Mux/1
  Sine Wave 0 rad/1 -> Saddle_Wave/1(A)
  Saddle_Wave/3(c) -> Mux/3
  Sine Wave -2/3pi rad/1 -> Saddle_Wave/2(B)
  Mux/1 -> Uref/1

== system model_sim_CHB5_36_new_temp/du//dt filter ==
  Series RLC Branch1 : powerlib/Elements/Series RLC Branch  LConnTagsString=__new0  RConnTagsString=__new0  BranchType=RC  Resistance=R_f  Inductance=L  SetiL0=off  InitialCurrent=0  Capacitance=C_f  Setx0=off  InitialVoltage=0  Measurements=None
  Series RLC Branch2 : powerlib/Elements/Series RLC Branch  LConnTagsString=__new0  RConnTagsString=__new0  BranchType=RC  Resistance=R_f  Inductance=L  SetiL0=off  InitialCurrent=0  Capacitance=C_f  Setx0=off  InitialVoltage=0  Measurements=None
  Series RLC Branch3 : powerlib/Elements/Series RLC Branch  LConnTagsString=__new0  RConnTagsString=__new0  BranchType=L  Resistance=R  Inductance=L_f  SetiL0=off  InitialCurrent=0  Capacitance=1e-6  Setx0=off  InitialVoltage=0  Measurements=None
  Series RLC Branch4 : powerlib/Elements/Series RLC Branch  LConnTagsString=__new0  RConnTagsString=__new0  BranchType=L  Resistance=R  Inductance=L_f  SetiL0=off  InitialCurrent=0  Capacitance=1e-6  Setx0=off  InitialVoltage=0  Measurements=None
  Series RLC Branch5 : powerlib/Elements/Series RLC Branch  LConnTagsString=__new0  RConnTagsString=__new0  BranchType=L  Resistance=R  Inductance=L_f  SetiL0=off  InitialCurrent=0  Capacitance=1e-6  Setx0=off  InitialVoltage=0  Measurements=None
  Series RLC Branch6 : powerlib/Elements/Series RLC Branch  LConnTagsString=__new0  RConnTagsString=__new0  BranchType=RC  Resistance=R_f  Inductance=L  SetiL0=off  InitialCurrent=0  Capacitance=C_f  Setx0=off  InitialVoltage=0  Measurements=None
  A : PMIOPort  Side=Left
  B : PMIOPort  Port=2  Side=Left
  C : PMIOPort  Port=3  Side=Left
  a : PMIOPort  Port=4  Side=Right
  b : PMIOPort  Port=5  Side=Right
  c : PMIOPort  Port=6  Side=Right
  connections:
  Series RLC Branch5/RConn1 -- C/RConn1
  Series RLC Branch6/LConn1 -- a/RConn1 -- Series RLC Branch3/LConn1
  Series RLC Branch5/LConn1 -- Series RLC Branch2/LConn1 -- c/RConn1
  Series RLC Branch2/RConn1 -- Series RLC Branch6/RConn1 -- Series RLC Branch1/RConn1
  Series RLC Branch1/LConn1 -- b/RConn1 -- Series RLC Branch4/LConn1
  Series RLC Branch4/RConn1 -- B/RConn1
  Series RLC Branch3/RConn1 -- A/RConn1

== system model_sim_CHB5_36_new_temp/pwm generator ==
  Uref : Inport
  pwm_en : Inport  Port=2
  Demux : Demux  Outputs=3
  NOT{1..6} (6 alike) : Logic  AllPortsSameDT=off  OutDataTypeStr=boolean
  Scope1 : Scope  NumInputPorts=4
  carrier : Subsystem
  pwm generator : Subsystem
  pwm generator1 : Subsystem
  pwm generator2 : Subsystem
  tag scope: pwm1=global, pwm2=global, pwm3=global, pwm4=global, pwm5=global, pwm6=global
  wires:
  pwm generator2/1(pwm_up) -> NOT2/1
  pwm generator2/2(pwm_down) -> NOT1/1
  pwm generator1/1(pwm_up) -> NOT4/1
  pwm generator1/2(pwm_down) -> NOT3/1
  pwm generator/1(pwm_up) -> NOT6/1
  pwm generator/2(pwm_down) -> NOT5/1
  Demux/1 -> Scope1/2, pwm generator/1(modulate_wave)
  Demux/2 -> pwm generator1/1(modulate_wave), Scope1/3
  Demux/3 -> Scope1/4, pwm generator2/1(modulate_wave)
  carrier/1(CARRIER_4*1) -> pwm generator2/2(Carrier_wave), pwm generator1/2(Carrier_wave), pwm generator/2(Carrier_wave), Scope1/1
  Uref/1 -> Demux/1
  NOT6/1 -> [pwm1]
  NOT5/1 -> [pwm2]
  NOT4/1 -> [pwm3]
  NOT3/1 -> [pwm4]
  NOT2/1 -> [pwm5]
  NOT1/1 -> [pwm6]
  pwm_en/1 -> NOT1/2, NOT2/2, NOT3/2, NOT4/2, NOT5/2, NOT6/2

== system model_sim_CHB5_36_new_temp/MAIN TOPOLOGY level-5/IGCT1 ==
  PWM : Inport
  Current Measurement1 : powerlib/Measurements/Current Measurement  PhasorSimulation=off  OutputType=Complex  PSBequivalent=0
  Demux : Demux
  Diode{1..3,6,8} (5 alike) : powerlib/Power Electronics/Diode  Ron=rto  Lon=0  Vf=vto  IC=0  UseSnubber=off  Rs=500  Cs=250e-9  Measurements=on
  IGBT{,1..3} (4 alike) : powerlib/Power Electronics/IGBT  Ron=rt  Lon=0  Vf=vt  Tf=1e-6  Tt=2e-6  IC=0  Rs=1e5  Cs=inf  Measurements=on
  Series RLC Branch1 : powerlib/Elements/Series RLC Branch  LConnTagsString=__new0  RConnTagsString=__new0  BranchType=RL  Resistance=1e-5  Inductance=3.0E-6  SetiL0=off  InitialCurrent=0  Capacitance=1e-6  Setx0=off  InitialVoltage=0  Measurements=None
  Series RLC Branch10 : powerlib/Elements/Series RLC Branch  LConnTagsString=__new0  RConnTagsString=__new0  BranchType=L  Resistance=1  Inductance=0.4e-6  SetiL0=off  InitialCurrent=0  Capacitance=1e-6  Setx0=off  InitialVoltage=0  Measurements=None
  Series RLC Branch12 : powerlib/Elements/Series RLC Branch  LConnTagsString=__new0  RConnTagsString=__new0  BranchType=RL  Resistance=1e-5  Inductance=1E-9  SetiL0=off  InitialCurrent=0  Capacitance=1e-6  Setx0=off  InitialVoltage=0  Measurements=None
  Series RLC Branch14 : powerlib/Elements/Series RLC Branch  LConnTagsString=__new0  RConnTagsString=__new0  BranchType=L  Resistance=1  Inductance=1E-7  SetiL0=off  InitialCurrent=0  Capacitance=1e-6  Setx0=off  InitialVoltage=0  Measurements=None
  Series RLC Branch2 : powerlib/Elements/Series RLC Branch  LConnTagsString=__new0  RConnTagsString=__new0  BranchType=RC  Resistance=1e-5  Inductance=20e-6  SetiL0=off  InitialCurrent=0  Capacitance=17e-6  Setx0=off  InitialVoltage=0  Measurements=None
  Series RLC Branch3 : powerlib/Elements/Series RLC Branch  LConnTagsString=__new0  RConnTagsString=__new0  BranchType=RL  Resistance=1e-5  Inductance=1E-9  SetiL0=off  InitialCurrent=0  Capacitance=1e-6  Setx0=off  InitialVoltage=0  Measurements=None
  Series RLC Branch5 : powerlib/Elements/Series RLC Branch  LConnTagsString=__new0  RConnTagsString=__new0  BranchType=L  Resistance=1  Inductance=1E-7  SetiL0=off  InitialCurrent=0  Capacitance=1e-6  Setx0=off  InitialVoltage=0  Measurements=None
  Series RLC Branch7 : powerlib/Elements/Series RLC Branch  LConnTagsString=__new0  RConnTagsString=__new0  BranchType=RL  Resistance=0.6  Inductance=1e-6  SetiL0=off  InitialCurrent=0  Capacitance=1e-6  Setx0=off  InitialVoltage=0  Measurements=None
  Series RLC Branch9 : powerlib/Elements/Series RLC Branch  LConnTagsString=__new0  RConnTagsString=__new0  BranchType=L  Resistance=1  Inductance=0.4e-6  SetiL0=off  InitialCurrent=0  Capacitance=1e-6  Setx0=off  InitialVoltage=0  Measurements=None
  Terminator{,1..9} (10 alike) : Terminator
  Udc+ : PMIOPort  Side=Left
  udc- : PMIOPort  Port=2  Side=Left
  p1 : PMIOPort  Port=3  Side=Right
  p2 : PMIOPort  Port=4  Side=Right
  wires:
  Diode3/1 -> Terminator9/1
  IGBT3/1 -> Terminator5/1
  [n1] -> IGBT3/1
  IGBT1/1 -> Terminator4/1
  IGBT2/1 -> Terminator3/1
  IGBT/1 -> Terminator2/1
  [n2] -> IGBT1/1
  [p1] -> IGBT2/1
  Current Measurement1/1 -> Terminator/1
  Diode2/1 -> Terminator8/1
  [p2] -> IGBT/1
  Diode8/1 -> Terminator7/1
  Diode1/1 -> Terminator6/1
  Diode6/1 -> Terminator1/1
  Demux/3 -> [n2]
  PWM/1 -> Demux/1
  Demux/1 -> [p2]
  Demux/2 -> [p1]
  Demux/4 -> [n1]
  connections:
  Series RLC Branch10/LConn1 -- udc-/RConn1
  Series RLC Branch9/LConn1 -- Udc+/RConn1
  Diode6/RConn1 -- Series RLC Branch7/RConn1 -- Series RLC Branch2/LConn1
  Current Measurement1/LConn1 -- Series RLC Branch1/RConn1 -- Series RLC Branch3/LConn1 -- Series RLC Branch12/LConn1
  Diode3/LConn1 -- IGBT3/RConn1 -- Series RLC Branch14/RConn1
  Series RLC Branch3/RConn1 -- IGBT/LConn1 -- Diode8/RConn1
  Diode1/LConn1 -- Series RLC Branch5/RConn1 -- IGBT1/RConn1
  Current Measurement1/RConn1 -- Diode6/LConn1
  Diode2/RConn1 -- Series RLC Branch12/RConn1 -- IGBT2/LConn1
  p1/RConn1 -- Diode2/LConn1 -- Diode3/RConn1 -- IGBT3/LConn1 -- IGBT2/RConn1
  Series RLC Branch5/LConn1 -- Series RLC Branch14/LConn1 -- Series RLC Branch10/RConn1 -- Series RLC Branch2/RConn1
  Series RLC Branch1/LConn1 -- Series RLC Branch7/LConn1 -- Series RLC Branch9/RConn1
  p2/RConn1 -- IGBT1/LConn1 -- Diode1/RConn1 -- Diode8/LConn1 -- IGBT/RConn1

== system model_sim_CHB5_36_new_temp/MAIN TOPOLOGY level-5/IGCT2 ==
  PWM : Inport
  Current Measurement1 : powerlib/Measurements/Current Measurement  PhasorSimulation=off  OutputType=Complex  PSBequivalent=0
  Demux : Demux
  Diode{1..3,6,8} (5 alike) : powerlib/Power Electronics/Diode  Ron=rto  Lon=0  Vf=vto  IC=0  UseSnubber=off  Rs=500  Cs=250e-9  Measurements=on
  IGBT{,1..3} (4 alike) : powerlib/Power Electronics/IGBT  Ron=rt  Lon=0  Vf=vt  Tf=1e-6  Tt=2e-6  IC=0  Rs=1e5  Cs=inf  Measurements=on
  Series RLC Branch1 : powerlib/Elements/Series RLC Branch  LConnTagsString=__new0  RConnTagsString=__new0  BranchType=RL  Resistance=1e-5  Inductance=3.0E-6  SetiL0=off  InitialCurrent=0  Capacitance=1e-6  Setx0=off  InitialVoltage=0  Measurements=None
  Series RLC Branch10 : powerlib/Elements/Series RLC Branch  LConnTagsString=__new0  RConnTagsString=__new0  BranchType=L  Resistance=1  Inductance=0.4e-6  SetiL0=off  InitialCurrent=0  Capacitance=1e-6  Setx0=off  InitialVoltage=0  Measurements=None
  Series RLC Branch12 : powerlib/Elements/Series RLC Branch  LConnTagsString=__new0  RConnTagsString=__new0  BranchType=RL  Resistance=1e-5  Inductance=1E-9  SetiL0=off  InitialCurrent=0  Capacitance=1e-6  Setx0=off  InitialVoltage=0  Measurements=None
  Series RLC Branch14 : powerlib/Elements/Series RLC Branch  LConnTagsString=__new0  RConnTagsString=__new0  BranchType=L  Resistance=1  Inductance=1E-7  SetiL0=off  InitialCurrent=0  Capacitance=1e-6  Setx0=off  InitialVoltage=0  Measurements=None
  Series RLC Branch2 : powerlib/Elements/Series RLC Branch  LConnTagsString=__new0  RConnTagsString=__new0  BranchType=RC  Resistance=1e-5  Inductance=20e-6  SetiL0=off  InitialCurrent=0  Capacitance=17e-6  Setx0=off  InitialVoltage=0  Measurements=None
  Series RLC Branch3 : powerlib/Elements/Series RLC Branch  LConnTagsString=__new0  RConnTagsString=__new0  BranchType=RL  Resistance=1e-5  Inductance=1E-9  SetiL0=off  InitialCurrent=0  Capacitance=1e-6  Setx0=off  InitialVoltage=0  Measurements=None
  Series RLC Branch5 : powerlib/Elements/Series RLC Branch  LConnTagsString=__new0  RConnTagsString=__new0  BranchType=L  Resistance=1  Inductance=1E-7  SetiL0=off  InitialCurrent=0  Capacitance=1e-6  Setx0=off  InitialVoltage=0  Measurements=None
  Series RLC Branch7 : powerlib/Elements/Series RLC Branch  LConnTagsString=__new0  RConnTagsString=__new0  BranchType=RL  Resistance=0.6  Inductance=1e-6  SetiL0=off  InitialCurrent=0  Capacitance=1e-6  Setx0=off  InitialVoltage=0  Measurements=None
  Series RLC Branch9 : powerlib/Elements/Series RLC Branch  LConnTagsString=__new0  RConnTagsString=__new0  BranchType=L  Resistance=1  Inductance=0.4e-6  SetiL0=off  InitialCurrent=0  Capacitance=1e-6  Setx0=off  InitialVoltage=0  Measurements=None
  Terminator{,1..9} (10 alike) : Terminator
  Udc+ : PMIOPort  Side=Left
  udc- : PMIOPort  Port=2  Side=Left
  p1 : PMIOPort  Port=3  Side=Right
  p2 : PMIOPort  Port=4  Side=Right
  wires:
  Demux/4 -> [n1]
  Demux/2 -> [p1]
  Demux/1 -> [p2]
  PWM/1 -> Demux/1
  Demux/3 -> [n2]
  Diode6/1 -> Terminator1/1
  Diode1/1 -> Terminator6/1
  Diode8/1 -> Terminator7/1
  [p2] -> IGBT/1
  Diode2/1 -> Terminator8/1
  Current Measurement1/1 -> Terminator/1
  [p1] -> IGBT2/1
  [n2] -> IGBT1/1
  IGBT/1 -> Terminator2/1
  IGBT2/1 -> Terminator3/1
  IGBT1/1 -> Terminator4/1
  [n1] -> IGBT3/1
  IGBT3/1 -> Terminator5/1
  Diode3/1 -> Terminator9/1
  connections:
  IGBT/RConn1 -- Diode8/LConn1 -- Diode1/RConn1 -- IGBT1/LConn1 -- p2/RConn1
  Series RLC Branch9/RConn1 -- Series RLC Branch7/LConn1 -- Series RLC Branch1/LConn1
  Series RLC Branch2/RConn1 -- Series RLC Branch10/RConn1 -- Series RLC Branch14/LConn1 -- Series RLC Branch5/LConn1
  IGBT2/RConn1 -- IGBT3/LConn1 -- Diode3/RConn1 -- Diode2/LConn1 -- p1/RConn1
  IGBT2/LConn1 -- Series RLC Branch12/RConn1 -- Diode2/RConn1
  Current Measurement1/RConn1 -- Diode6/LConn1
  IGBT1/RConn1 -- Series RLC Branch5/RConn1 -- Diode1/LConn1
  Diode8/RConn1 -- IGBT/LConn1 -- Series RLC Branch3/RConn1
  Series RLC Branch14/RConn1 -- IGBT3/RConn1 -- Diode3/LConn1
  Series RLC Branch12/LConn1 -- Series RLC Branch3/LConn1 -- Series RLC Branch1/RConn1 -- Current Measurement1/LConn1
  Series RLC Branch2/LConn1 -- Series RLC Branch7/RConn1 -- Diode6/RConn1
  Series RLC Branch9/LConn1 -- Udc+/RConn1
  Series RLC Branch10/LConn1 -- udc-/RConn1

== system model_sim_CHB5_36_new_temp/MAIN TOPOLOGY level-5/IGCT3 ==
  PWM : Inport
  Current Measurement1 : powerlib/Measurements/Current Measurement  PhasorSimulation=off  OutputType=Complex  PSBequivalent=0
  Demux : Demux
  Diode{1..3,6,8} (5 alike) : powerlib/Power Electronics/Diode  Ron=rto  Lon=0  Vf=vto  IC=0  UseSnubber=off  Rs=500  Cs=250e-9  Measurements=on
  IGBT{,1..3} (4 alike) : powerlib/Power Electronics/IGBT  Ron=rt  Lon=0  Vf=vt  Tf=1e-6  Tt=2e-6  IC=0  Rs=1e5  Cs=inf  Measurements=on
  Series RLC Branch1 : powerlib/Elements/Series RLC Branch  LConnTagsString=__new0  RConnTagsString=__new0  BranchType=RL  Resistance=1e-5  Inductance=3.0E-6  SetiL0=off  InitialCurrent=0  Capacitance=1e-6  Setx0=off  InitialVoltage=0  Measurements=None
  Series RLC Branch10 : powerlib/Elements/Series RLC Branch  LConnTagsString=__new0  RConnTagsString=__new0  BranchType=L  Resistance=1  Inductance=0.4e-6  SetiL0=off  InitialCurrent=0  Capacitance=1e-6  Setx0=off  InitialVoltage=0  Measurements=None
  Series RLC Branch12 : powerlib/Elements/Series RLC Branch  LConnTagsString=__new0  RConnTagsString=__new0  BranchType=RL  Resistance=1e-5  Inductance=1E-9  SetiL0=off  InitialCurrent=0  Capacitance=1e-6  Setx0=off  InitialVoltage=0  Measurements=None
  Series RLC Branch14 : powerlib/Elements/Series RLC Branch  LConnTagsString=__new0  RConnTagsString=__new0  BranchType=L  Resistance=1  Inductance=1E-7  SetiL0=off  InitialCurrent=0  Capacitance=1e-6  Setx0=off  InitialVoltage=0  Measurements=None
  Series RLC Branch2 : powerlib/Elements/Series RLC Branch  LConnTagsString=__new0  RConnTagsString=__new0  BranchType=RC  Resistance=1e-5  Inductance=20e-6  SetiL0=off  InitialCurrent=0  Capacitance=17e-6  Setx0=off  InitialVoltage=0  Measurements=None
  Series RLC Branch3 : powerlib/Elements/Series RLC Branch  LConnTagsString=__new0  RConnTagsString=__new0  BranchType=RL  Resistance=1e-5  Inductance=1E-9  SetiL0=off  InitialCurrent=0  Capacitance=1e-6  Setx0=off  InitialVoltage=0  Measurements=None
  Series RLC Branch5 : powerlib/Elements/Series RLC Branch  LConnTagsString=__new0  RConnTagsString=__new0  BranchType=L  Resistance=1  Inductance=1E-7  SetiL0=off  InitialCurrent=0  Capacitance=1e-6  Setx0=off  InitialVoltage=0  Measurements=None
  Series RLC Branch7 : powerlib/Elements/Series RLC Branch  LConnTagsString=__new0  RConnTagsString=__new0  BranchType=RL  Resistance=0.6  Inductance=1e-6  SetiL0=off  InitialCurrent=0  Capacitance=1e-6  Setx0=off  InitialVoltage=0  Measurements=None
  Series RLC Branch9 : powerlib/Elements/Series RLC Branch  LConnTagsString=__new0  RConnTagsString=__new0  BranchType=L  Resistance=1  Inductance=0.4e-6  SetiL0=off  InitialCurrent=0  Capacitance=1e-6  Setx0=off  InitialVoltage=0  Measurements=None
  Terminator{,1..9} (10 alike) : Terminator
  Udc+ : PMIOPort  Side=Left
  udc- : PMIOPort  Port=2  Side=Left
  p1 : PMIOPort  Port=3  Side=Right
  p2 : PMIOPort  Port=4  Side=Right
  wires:
  Demux/4 -> [n1]
  Demux/2 -> [p1]
  Demux/1 -> [p2]
  PWM/1 -> Demux/1
  Demux/3 -> [n2]
  Diode6/1 -> Terminator1/1
  Diode1/1 -> Terminator6/1
  Diode8/1 -> Terminator7/1
  [p2] -> IGBT/1
  Diode2/1 -> Terminator8/1
  Current Measurement1/1 -> Terminator/1
  [p1] -> IGBT2/1
  [n2] -> IGBT1/1
  IGBT/1 -> Terminator2/1
  IGBT2/1 -> Terminator3/1
  IGBT1/1 -> Terminator4/1
  [n1] -> IGBT3/1
  IGBT3/1 -> Terminator5/1
  Diode3/1 -> Terminator9/1
  connections:
  IGBT/RConn1 -- Diode8/LConn1 -- Diode1/RConn1 -- IGBT1/LConn1 -- p2/RConn1
  Series RLC Branch9/RConn1 -- Series RLC Branch7/LConn1 -- Series RLC Branch1/LConn1
  Series RLC Branch2/RConn1 -- Series RLC Branch10/RConn1 -- Series RLC Branch14/LConn1 -- Series RLC Branch5/LConn1
  IGBT2/RConn1 -- IGBT3/LConn1 -- Diode3/RConn1 -- Diode2/LConn1 -- p1/RConn1
  IGBT2/LConn1 -- Series RLC Branch12/RConn1 -- Diode2/RConn1
  Current Measurement1/RConn1 -- Diode6/LConn1
  IGBT1/RConn1 -- Series RLC Branch5/RConn1 -- Diode1/LConn1
  Diode8/RConn1 -- IGBT/LConn1 -- Series RLC Branch3/RConn1
  Series RLC Branch14/RConn1 -- IGBT3/RConn1 -- Diode3/LConn1
  Series RLC Branch12/LConn1 -- Series RLC Branch3/LConn1 -- Series RLC Branch1/RConn1 -- Current Measurement1/LConn1
  Series RLC Branch2/LConn1 -- Series RLC Branch7/RConn1 -- Diode6/RConn1
  Series RLC Branch9/LConn1 -- Udc+/RConn1
  Series RLC Branch10/LConn1 -- udc-/RConn1
